simulink model "s_kalm3"  (Simulink 4.00)
settings: Solver=ode45  SolverMode=SingleTasking  StartTime=0.0  StopTime=200  MaxStep=0.10  RelTol=1e-3  AbsTol=1e-6
values from neighbouring files (symbols this model uses):
  dt = 0.1    [estimate_1.m]    (also in estimate_2.m; estimate_3.m; estimate_31.m; kalm1.m)
  qv = 0.2    [kalm1.m]    (also in kalm2.m; kalm3.m = 0.02)
  qw = 0.1    [kalm1.m]    (also in kalm2.m; kalm3.m; kalm4.m = 0.01)
  Ts = 0.5    [abeob1.m]    (also in akalm1.m = 0.25; alqrd1.m = 0.25; kalm2.m; kalm3.m)
undefined symbols (not defined in the file or in its folder): ns
settings Model: LastModifiedBy=Administrator  SaveTime=off  SaveOutput=off  LimitDataPoints=off  BlockReductionOpt=off

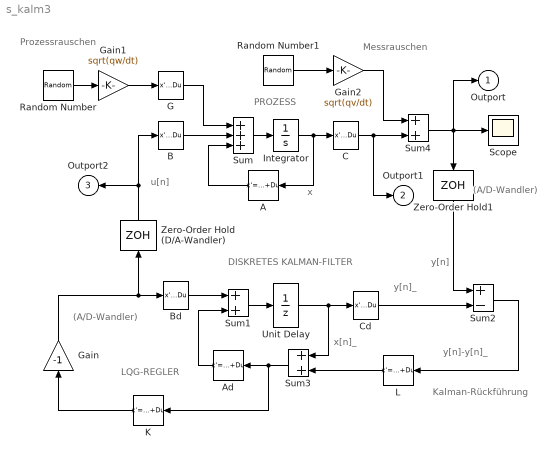
== system s_kalm3 ==
  note: (A/D-Wandler)
  note: LQG-REGLER
  note: Kalman-Rückführung
  note: DISKRETES KALMAN-FILTER
  note: (A/D-Wandler)
  note: x[n]_
  note: x
  note: y[n]
  note: y[n]_
  note: u[n]
  note: y[n]-y[n]_
  note: Prozessrauschen
  note: PROZESS
  note: Messrauschen
  A : StateSpace  Orientation=left  A=[]  B=[]  C=[]  D=K  X0=0  Realization=auto  AbsoluteTolerance=auto  mask(Matrix Gain){@1=A}
      mask prompts: @1 "Gain matrix:"
      mask help: Matrix Gain.
      mask init:
      | K = @1;
      mask Help: Multiplies input vector by entered matrix to produce output vector (y=Au).
      mask Display: disp('K')
  Ad : StateSpace  Orientation=left  A=[]  B=[]  C=[]  D=K  X0=0  Realization=auto  AbsoluteTolerance=auto  mask(Matrix Gain){@1=Ad}
      mask prompts: @1 "Gain matrix:"
      mask help: Matrix Gain.
      mask init:
      | K = @1;
      mask Help: Multiplies input vector by entered matrix to produce output vector (y=Au).
      mask Display: disp('K')
  B : StateSpace  A=[]  B=[]  C=[]  D=K  X0=0  Realization=auto  AbsoluteTolerance=auto  mask(Matrix Gain){@1=B}
      mask prompts: @1 "Gain matrix:"
      mask help: Matrix Gain.
      mask init:
      | K = @1;
      mask Help: Multiplies input vector by entered matrix to produce output vector (y=Au).
      mask Display: disp('K')
  Bd : StateSpace  A=[]  B=[]  C=[]  D=K  X0=0  Realization=auto  AbsoluteTolerance=auto  mask(Matrix Gain){@1=Bd}
      mask prompts: @1 "Gain matrix:"
      mask help: Matrix Gain.
      mask init:
      | K = @1;
      mask Help: Multiplies input vector by entered matrix to produce output vector (y=Au).
      mask Display: disp('K')
  C : StateSpace  A=[]  B=[]  C=[]  D=K  X0=0  Realization=auto  AbsoluteTolerance=auto  mask(Matrix Gain){@1=C}
      mask prompts: @1 "Gain matrix:"
      mask help: Matrix Gain.
      mask init:
      | K = @1;
      mask Help: Multiplies input vector by entered matrix to produce output vector (y=Au).
      mask Display: disp('K')
  Cd : StateSpace  A=[]  B=[]  C=[]  D=K  X0=0  Realization=auto  AbsoluteTolerance=auto  mask(Matrix Gain){@1=Cd}
      mask prompts: @1 "Gain matrix:"
      mask help: Matrix Gain.
      mask init:
      | K = @1;
      mask Help: Multiplies input vector by entered matrix to produce output vector (y=Au).
      mask Display: disp('K')
  G : StateSpace  A=[]  B=[]  C=[]  D=K  X0=0  Realization=auto  AbsoluteTolerance=auto  mask(Matrix Gain){@1=G}
      mask prompts: @1 "Gain matrix:"
      mask help: Matrix Gain.
      mask init:
      | K = @1;
      mask Help: Multiplies input vector by entered matrix to produce output vector (y=Au).
      mask Display: disp('K')
  Gain : Gain  Orientation=up  Gain=-1  Multiplication=Element-wise(K.*u)  SaturateOnIntegerOverflow=on
  Gain1 : Gain  Gain=sqrt(qw/dt)  Multiplication=Element-wise(K.*u)  SaturateOnIntegerOverflow=on
  Gain2 : Gain  Gain=sqrt(qv/dt)  Multiplication=Element-wise(K.*u)  SaturateOnIntegerOverflow=on
  Integrator : Integrator  ExternalReset=none  InitialConditionSource=internal  InitialCondition=[1 2 1 -2 1 2]  LimitOutput=off  UpperSaturationLimit=inf  LowerSaturationLimit=-inf  ShowSaturationPort=off  ShowStatePort=off  AbsoluteTolerance=auto
  K : StateSpace  Orientation=left  A=[]  B=[]  C=[]  D=K  X0=0  Realization=auto  AbsoluteTolerance=auto  mask(Matrix Gain){@1=K}
      mask prompts: @1 "Gain matrix:"
      mask help: Matrix Gain.
      mask init:
      | K = @1;
      mask Help: Multiplies input vector by entered matrix to produce output vector (y=Au).
      mask Display: disp('K')
  L : StateSpace  Orientation=left  A=[]  B=[]  C=[]  D=K  X0=0  Realization=auto  AbsoluteTolerance=auto  mask(Matrix Gain){@1=L}
      mask prompts: @1 "Gain matrix:"
      mask help: Matrix Gain.
      mask init:
      | K = @1;
      mask Help: Multiplies input vector by entered matrix to produce output vector (y=Au).
      mask Display: disp('K')
  Random Number : RandomNumber  Mean=zeros(1,ns)  Variance=ones(1,ns)  Seed=rand(1,ns)*259  SampleTime=0
  Random Number1 : RandomNumber  Mean=0  Variance=1  Seed=15389  SampleTime=0
  Scope : Scope
      settings: TickLabels=on  TimeRange=5.140000  YMin=-16.281600  YMax=16.281600  SaveToWorkspace=off  SaveName=ScopeData  DataFormat=Array  LimitDataPoints=on  MaxDataPoints=5000
  Sum : Sum  Inputs=+++  SaturateOnIntegerOverflow=on
  Sum1 : Sum  Inputs=++  SaturateOnIntegerOverflow=on
  Sum2 : Sum  Inputs=+-  SaturateOnIntegerOverflow=on
  Sum3 : Sum  Orientation=left  Inputs=++  SaturateOnIntegerOverflow=on
  Sum4 : Sum  Inputs=++  SaturateOnIntegerOverflow=on
  Unit Delay : UnitDelay  X0=0  SampleTime=Ts
  "Zero-Order Hold (D/A-Wandler) " : ZeroOrderHold  Orientation=up  SampleTime=Ts
  Zero-Order Hold1 : ZeroOrderHold  Orientation=down  SampleTime=Ts
  Outport : Outport  Port=1  InitialOutput=0
  Outport1 : Outport  Port=2  InitialOutput=0
  Outport2 : Outport  Orientation=left  Port=3  InitialOutput=0
  wires:
  Gain/1 -> Bd/1, "Zero-Order Hold (D/A-Wandler) "/1
  K/1 -> Gain/1
  Sum3/1 -> K/1, Ad/1
  Bd/1 -> Sum1/1
  L/1 -> Sum3/2
  Unit Delay/1 -> Sum3/1, Cd/1
  Sum2/1 -> L/1
  Zero-Order Hold1/1 -> Sum2/1
  Sum4/1 -> Scope/1, Zero-Order Hold1/1, Outport/1
  C/1 -> Outport1/1, Sum4/2
  Gain1/1 -> G/1
  G/1 -> Sum/1
  Gain2/1 -> Sum4/1
  A/1 -> Sum/3
  B/1 -> Sum/2
  Cd/1 -> Sum2/2
  Ad/1 -> Sum1/2
  Sum1/1 -> Unit Delay/1
  Integrator/1 -> C/1, A/1
  Sum/1 -> Integrator/1
  Random Number/1 -> Gain1/1
  Random Number1/1 -> Gain2/1
  "Zero-Order Hold (D/A-Wandler) "/1 -> B/1, Outport2/1
